simulink model "model"  (R2016b)
settings: Solver=VariableStepAuto  StartTime=0.0  StopTime=200.0  RelTol=1e-3
libraries: fuzblock x1
settings Model: Creator=novo  LastModifiedBy=jani

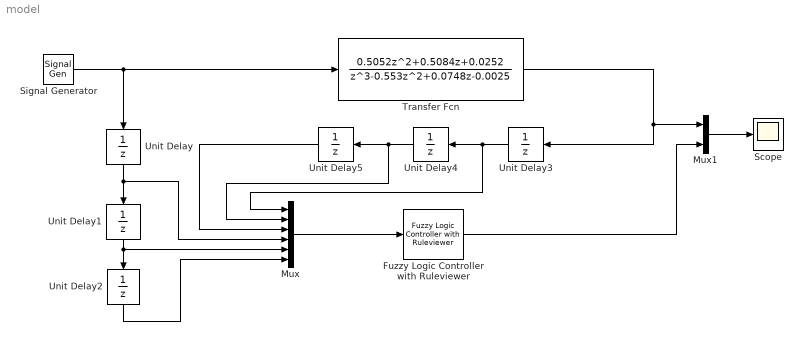
== system model ==
  Fuzzy Logic Controller with Ruleviewer : fuzblock/Fuzzy Logic  Controller  with Ruleviewer  fismatrix=fcmfis  Ts=1
  Mux : Mux  Inputs=6
  Mux1 : Mux  Inputs=2
  Scope : Scope
  Signal Generator : SignalGenerator  Frequency=0.1  Units=rad/sec
  Transfer Fcn : DiscreteTransferFcn  Numerator="[0       0.5052    0.5084    0.0252]"  Denominator="[1 -0.553    0.0748   -0.0025]"
  Unit Delay{,1..5} (6 alike) : UnitDelay  SampleTime=0.2
  wires:
  Signal Generator/1 -> Transfer Fcn/1, Unit Delay/1
  Transfer Fcn/1 -> Unit Delay3/1, Mux1/1
  Unit Delay/1 -> Unit Delay1/1, Mux/4
  Unit Delay1/1 -> Mux/5, Unit Delay2/1
  Unit Delay2/1 -> Mux/6
  Unit Delay3/1 -> Unit Delay4/1, Mux/1
  Unit Delay4/1 -> Mux/2, Unit Delay5/1
  Unit Delay5/1 -> Mux/3
  Mux/1 -> Fuzzy Logic Controller with Ruleviewer/1
  Fuzzy Logic Controller with Ruleviewer/1 -> Mux1/2
  Mux1/1 -> Scope/1
